simulink model "untitled1"  (Simulink 7.4)
settings: Solver=ode45  StartTime=0.0  StopTime=5.0  RelTol=1e-3
settings Model: Creator=bukova.2018  LastModifiedBy=bukova.2018

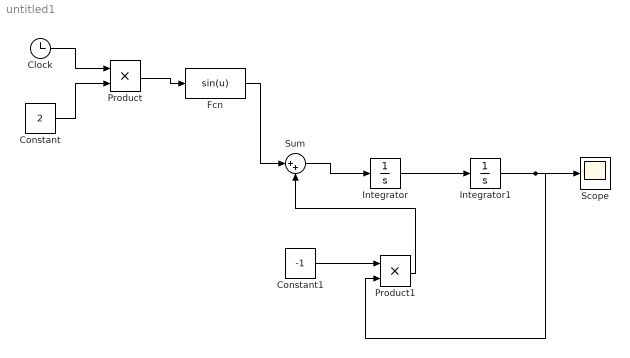
== system untitled1 ==
  Clock : Clock
      settings: Decimation=10
  Constant : Constant  Value=2  OutDataType=fixdt(1, 16)  OutScaling=2^0
  Constant1 : Constant  Value=-1  OutDataType=fixdt(1, 16)  OutScaling=2^0
  Fcn : Fcn  Expr=sin(u)
  Integrator : Integrator
  Integrator1 : Integrator
  Product : Product  OutDataType=fixdt(1, 16)  OutScaling=2^0  RndMeth=Zero
  Product1 : Product  OutDataType=fixdt(1, 16)  OutScaling=2^0  RndMeth=Zero
  Scope : Scope
  Sum : Sum  Inputs=|++  OutDataType=fixdt(1, 16)  OutScaling=2^0
  wires:
  Constant/1 -> Product/2
  Clock/1 -> Product/1
  Product/1 -> Fcn/1
  Fcn/1 -> Sum/1
  Sum/1 -> Integrator/1
  Integrator/1 -> Integrator1/1
  Integrator1/1 -> Scope/1, Product1/2
  Constant1/1 -> Product1/1
  Product1/1 -> Sum/2
